simulink model "Resp18e_updatedPulse"  (Simulink 7.3)
settings: Solver=ode23  StartTime=0.0  StopTime=20  FixedStep=0.01  MaxStep=0.05  RelTol=1e-6
values from neighbouring files (symbols this model uses):
  alpha_CO2_brain = 2.9/1e3*760/P_stp/K_stp    (= 0.00097047576489)    [initialize_parameters.m]
  alpha_CO2_fat = 0.9/K_stp/P_stp    (= 0.000396292281489)    [initialize_parameters.m]
  alpha_CO2_heart = 2.4/1e3*760/P_stp/K_stp    (= 0.00080315235715)    [initialize_parameters.m]
  alpha_CO2_lean = 4.2/1e3*760/P_stp/K_stp    (= 0.00140551662501)    [initialize_parameters.m]
  alpha_CO2_lungtiss_fast = alpha_CO2_lungtiss_fast./0.1333    [initialize_parameters.m]
  alpha_CO2_muscle = 4.2/1e3*760/P_stp/K_stp    (= 0.00140551662501)    [initialize_parameters.m]
  alpha_CO2_other = 3.0/1e3*760/P_stp/K_stp    (= 0.00100394044644)    [initialize_parameters.m]
  alpha_O2_fat = 5*0.024/K_stp/P_stp    (= 5.28389708651e-05)    [initialize_parameters.m]
  alpha_O2_tissue = 0.024/K_stp/P_stp    (= 1.0567794173e-05)    [initialize_parameters.m]
  BOHRF0 = O2_SHIFT - T_BLOOD_M_37 * (0.024 + BOHRF * 0.0147) - BOHRF1 * 7.4    (= -3.552)    [initialize_parameters.m]
  BOHRF1 = BOHRF * (1 - T_BLOOD_M_37 * 0.0065)    (= 0.48)    [initialize_parameters.m]
  C_a_CO2_i = 20.8e-3    (= 0.0208)    [initialize_parameters.m]    (also in resp18e_ic_norm.mat = 0.0202734801806)
  C_a_O2_i = 8.95e-3    (= 0.00895)    [initialize_parameters.m]    (also in resp18e_ic_norm.mat = 0.00918087581167)
  CAP_O2 = 0.01 * CAP_O2    (= 0.201)    [initialize_parameters.m]
  Cardiac_duty_cycle = 40    [initialize_parameters.m]
  Co_CO2_brain = 401*K_Co_CO2/1e3/K_stp    (= 0.0107345869894)    [initialize_parameters.m]
  Co_CO2_heart = 487*K_Co_CO2/1e3/K_stp    (= 0.0130367677403)    [initialize_parameters.m]
  Co_CO2_lean = 342*K_Co_CO2/1e3/K_stp    (= 0.00915518391618)    [initialize_parameters.m]
  Co_CO2_muscle = 342*K_Co_CO2/1e3/K_stp    (= 0.00915518391618)    [initialize_parameters.m]
  Co_CO2_other = 355*K_Co_CO2/1e3/K_stp    (= 0.00950318798317)    [initialize_parameters.m]
  DH2ODS = DH2ODS + 0.007 * HB_MEQ * (HB_MEQ - 9) / (13.5 * (13.5 - 9))    (= 0.00498709726946)    [initialize_parameters.m]
  F_insp_alv_alvds = F_v_alv_deadspace / F_insp_hivq    (= 0.00299401197605)    [initialize_parameters.m]
  F_insp_alv_hivq = F_v_alv_hivq      / F_insp_hivq    (= 0.997005988024)    [initialize_parameters.m]
  F_insp_alv_lovq = F_v_alv_lovq      / F_insp_lovq    (= 0.5)    [initialize_parameters.m]
  F_insp_alv_midvq = F_v_alv_midvq     / F_insp_lovq    (= 0.5)    [initialize_parameters.m]
  F_insp_hivq = F_v_alv_deadspace + F_v_alv_hivq    (= 0.334)    [initialize_parameters.m]
  F_insp_lovq = F_v_alv_midvq     + F_v_alv_lovq    (= 0.666)    [initialize_parameters.m]
  Fi_CO2_param_est = 0.01    [initialize_parameters.m]
  Fi_error = 1e-6    (= 1e-06)    [initialize_parameters.m]
  Fi_N2_mean = 1-(Fi_O2_mean + Fi_N2O_mean)    (= 0.65)    [initialize_parameters.m]
  Fi_O2_mean = 0.35    [initialize_parameters.m]
  Fi_O2_param_est = 0.01    [initialize_parameters.m]
  Fq_brain = 0.114    [initialize_parameters.m]
  Fq_error = 1e-8    (= 1e-08)    [initialize_parameters.m]
  Fq_fat = 0.103    [initialize_parameters.m]
  Fq_heart = 0.041    [initialize_parameters.m]
  Fq_hepatic = 0.069    [initialize_parameters.m]
  Fq_kidneys = 0.215    [initialize_parameters.m]
  Fq_lean = 0.090    (= 0.09)    [initialize_parameters.m]
  Fq_lungs_anatomicalshunt = 0.01    [initialize_parameters.m]
  Fq_lungs_hivq = (1-Fq_lungs_pulmshunt-Fq_lungs_anatomicalshunt)    *F_v_alv_hivq/(F_v_alv_hivq+F_v_alv_midvq+F_v_alv_lovq)    (= 0.3)    [initialize_parameters.m]
  Fq_lungs_lovq = (1-Fq_lungs_pulmshunt-Fq_lungs_anatomicalshunt)    *F_v_alv_lovq/(F_v_alv_hivq+F_v_alv_midvq+F_v_alv_lovq)    (= 0.3)    [initialize_parameters.m]
  Fq_lungs_midvq = (1-Fq_lungs_pulmshunt-Fq_lungs_anatomicalshunt)    *F_v_alv_midvq/(F_v_alv_hivq+F_v_alv_midvq+F_v_alv_lovq)    (= 0.3)    [initialize_parameters.m]
  Fq_lungs_pulmshunt = 0.09    [initialize_parameters.m]
  Fq_muscle = 0.096    [initialize_parameters.m]
  Fq_pershunt = 0.101    [initialize_parameters.m]
  Fq_portal = 0.171    [initialize_parameters.m]
  FRC = 2.2    [initialize_parameters.m]
  H2OB = H2OVC + 0.938 * (1 - VC_74)    (= 0.840191964286)    [initialize_parameters.m]
  k_CO2_lungtiss_fast_alvds = k_CO2_lungtiss_fast*F_v_alv_deadspace    (= 3.63090772693e-07)    [initialize_parameters.m]
  k_CO2_lungtiss_fast_hivq = k_CO2_lungtiss_fast*F_v_alv_hivq    (= 0.000120909227307)    [initialize_parameters.m]
  k_CO2_lungtiss_fast_lovq = k_CO2_lungtiss_fast*F_v_alv_lovq    (= 0.000120909227307)    [initialize_parameters.m]
  k_CO2_lungtiss_fast_midvq = k_CO2_lungtiss_fast*F_v_alv_midvq    (= 0.000120909227307)    [initialize_parameters.m]
  k_CO2_lungtiss_slow_alvds = k_CO2_lungtiss_slow*F_v_alv_deadspace    (= 4.95123780945e-09)    [initialize_parameters.m]
  k_CO2_lungtiss_slow_hivq = k_CO2_lungtiss_slow*F_v_alv_hivq    (= 1.64876219055e-06)    [initialize_parameters.m]
  k_CO2_lungtiss_slow_lovq = k_CO2_lungtiss_slow*F_v_alv_lovq    (= 1.64876219055e-06)    [initialize_parameters.m]
  k_CO2_lungtiss_slow_midvq = k_CO2_lungtiss_slow*F_v_alv_midvq    (= 1.64876219055e-06)    [initialize_parameters.m]
  K_diff_CO2_hivq = K_diff_CO2*F_v_alv_hivq    (= 0.0014985)    [initialize_parameters.m]
  K_diff_CO2_lovq = K_diff_CO2*F_v_alv_lovq    (= 0.0014985)    [initialize_parameters.m]
  K_diff_CO2_midvq = K_diff_CO2*F_v_alv_midvq    (= 0.0014985)    [initialize_parameters.m]
  K_diff_O2_hivq = K_diff_O2*F_v_alv_hivq    (= 7.326e-05)    [initialize_parameters.m]
  K_diff_O2_lovq = K_diff_O2*F_v_alv_lovq    (= 7.326e-05)    [initialize_parameters.m]
  K_diff_O2_midvq = K_diff_O2*F_v_alv_midvq    (= 7.326e-05)    [initialize_parameters.m]
  K_exp_alv_alvds = 1/1    (= 1)    [initialize_parameters.m]
  K_exp_alv_hivq = 1/1    (= 1)    [initialize_parameters.m]
  K_press = 760/101.325    (= 7.50061682704)    [initialize_parameters.m]
  K_stp = R*(T_stp+273.15)/(P_stp*1000)    (= 22.4135311621)    [initialize_parameters.m]
  Kg_alv = R*(T_alv+273.15)/(P_baro*1000)    (= 25.3668469802)    [initialize_parameters.m]
  LN10 = 2.30258509299405    (= 2.30258509299)    [initialize_parameters.m]
  m_alv_alvds_i = (FRC-V_deadspace_total)/Kg_alv * F_v_alv_deadspace    [initialize_parameters.m]
  m_alv_hivq_i = (FRC-V_deadspace_total)/Kg_alv * F_v_alv_hivq    [initialize_parameters.m]
  m_alv_lovq_i = (FRC-V_deadspace_total)/Kg_alv * F_v_alv_lovq    [initialize_parameters.m]
  m_alv_midvq_i = (FRC-V_deadspace_total)/Kg_alv * F_v_alv_midvq    [initialize_parameters.m]
  m_CO2_alv_alvds_i = F_CO2_i * m_alv_alvds_i    [initialize_parameters.m]
  m_CO2_alv_hivq_i = F_CO2_i * m_alv_hivq_i    [initialize_parameters.m]
  m_CO2_alv_lovq_i = F_CO2_i * m_alv_lovq_i    [initialize_parameters.m]
  m_CO2_alv_midvq_i = F_CO2_i * m_alv_midvq_i    [initialize_parameters.m]
  m_CO2_brain_b_i = C_a_CO2_i*Vb_brain    (= 0.002184)    [initialize_parameters.m]
  m_CO2_brain_t_i = (Co_CO2_brain  + alpha_CO2_brain *P_v_CO2_i)* Vt_brain    (= 0.0171268217946)    [initialize_parameters.m]
  m_CO2_common_b_i = C_a_CO2_i*Vb_common    (= 0.0170421333333)    [initialize_parameters.m]
  m_CO2_ds0_i = F_CO2_i*m_ds0_i    (= 0.000985538329597)    [initialize_parameters.m]
  m_CO2_ds_large_i = F_CO2_i * m_deadspace_large_1    [initialize_parameters.m]
  m_CO2_ds_med_hivq1_i = F_CO2_i * m_deadspace_med_hivq_1    [initialize_parameters.m]
  m_CO2_ds_med_hivq2_i = F_CO2_i * m_deadspace_med_hivq_2    [initialize_parameters.m]
  m_CO2_ds_med_lovq1_i = F_CO2_i * m_deadspace_med_lovq_1    [initialize_parameters.m]
  m_CO2_ds_med_lovq2_i = F_CO2_i * m_deadspace_med_lovq_2    [initialize_parameters.m]
  m_CO2_ds_small_alvds_i = F_CO2_i * m_deadspace_small_alvdeadspace    [initialize_parameters.m]
  m_CO2_ds_small_hivq_i = F_CO2_i * m_deadspace_small_hivq    [initialize_parameters.m]
  m_CO2_ds_small_lovq_i = F_CO2_i * m_deadspace_small_lovq    [initialize_parameters.m]
  m_CO2_ds_small_midvq_i = F_CO2_i * m_deadspace_small_midvq    [initialize_parameters.m]
  m_CO2_fat_b_i = C_a_CO2_i*Vb_fat    (= 0.0116896)    [initialize_parameters.m]
  m_CO2_fat_t_i = P_a_CO2_i*alpha_CO2_fat*Vt_fat    (= 0.0302752719501)    [initialize_parameters.m]
  m_CO2_heart_b_i = C_a_CO2_i*Vb_heart    (= 0.000832)    [initialize_parameters.m]
  m_CO2_heart_t_i = (Co_CO2_heart  + alpha_CO2_heart *P_v_CO2_i)* Vt_heart    (= 0.00402544335149)    [initialize_parameters.m]
  m_CO2_hepatic_b_i = C_a_CO2_i*Vb_hepatic    (= 0.0019136)    [initialize_parameters.m]
  m_CO2_kidneys_b_i = C_a_CO2_i*Vb_kidneys    (= 0.0012064)    [initialize_parameters.m]
  m_CO2_kidneys_t_i = (Co_CO2_other  + alpha_CO2_other *P_v_CO2_i)* Vt_kidneys    (= 0.0045902552907)    [initialize_parameters.m]
  m_CO2_lean_b_i = C_a_CO2_i*Vb_lean    (= 0.0191984)    [initialize_parameters.m]
  m_CO2_lean_t_i = (Co_CO2_lean   + alpha_CO2_lean  *P_v_CO2_i)* Vt_lean    (= 0.0884995401953)    [initialize_parameters.m]
  m_CO2_liver_t_i = (Co_CO2_other  + alpha_CO2_other *P_v_CO2_i)* Vt_liver    (= 0.0187019339777)    [initialize_parameters.m]
  m_CO2_lungtiss_fast_alvds_i = F_CO2_i*(P_baro-P_A_H2O)*V_lungtiss_alvds *alpha_CO2_lungtiss_fast(2)    [initialize_parameters.m]
  m_CO2_lungtiss_fast_hivq_i = F_CO2_i*(P_baro-P_A_H2O)*V_lungtiss_hivq  *alpha_CO2_lungtiss_fast(2)    [initialize_parameters.m]
  m_CO2_lungtiss_fast_lovq_i = F_CO2_i*(P_baro-P_A_H2O)*V_lungtiss_lovq  *alpha_CO2_lungtiss_fast(2)    [initialize_parameters.m]
  m_CO2_lungtiss_fast_midvq_i = F_CO2_i*(P_baro-P_A_H2O)*V_lungtiss_midvq *alpha_CO2_lungtiss_fast(2)    [initialize_parameters.m]
  m_CO2_lungtiss_slow_alvds_i = F_CO2_i*(P_baro-P_A_H2O)*V_lungtiss_alvds*alpha_CO2_lungtiss_slow    [initialize_parameters.m]
  m_CO2_lungtiss_slow_hivq_i = F_CO2_i*(P_baro-P_A_H2O)*V_lungtiss_hivq *alpha_CO2_lungtiss_slow    [initialize_parameters.m]
  m_CO2_lungtiss_slow_lovq_i = F_CO2_i*(P_baro-P_A_H2O)*V_lungtiss_lovq *alpha_CO2_lungtiss_slow    [initialize_parameters.m]
  m_CO2_lungtiss_slow_midvq_i = F_CO2_i*(P_baro-P_A_H2O)*V_lungtiss_midvq*alpha_CO2_lungtiss_slow    [initialize_parameters.m]
  m_CO2_LV_b_i = C_a_CO2_i*Vb_LV    (= 0.00391733333333)    [initialize_parameters.m]
  m_CO2_muscle_b_i = C_a_CO2_i*Vb_muscle    (= 0.0201344)    [initialize_parameters.m]
  m_CO2_muscle_t_i = (Co_CO2_muscle + alpha_CO2_muscle*P_v_CO2_i)* Vt_muscle    (= 0.363660431061)    [initialize_parameters.m]
  m_CO2_pershunt_b_i = C_a_CO2_i*Vb_pershunt    (= 0.0027248)    [initialize_parameters.m]
  m_CO2_portal_b_i = C_a_CO2_i*Vb_portal    (= 0.0210912)    [initialize_parameters.m]
  m_CO2_portal_t_i = (Co_CO2_other  + alpha_CO2_other *P_v_CO2_i)* Vt_portal    (= 0.0164739329706)    [initialize_parameters.m]
  m_CO2_pulmcap_b_hivq_i = C_a_CO2_i*Vb_pulmcap_hivq    (= 0.000630933333333)    [initialize_parameters.m]
  m_CO2_pulmcap_b_lovq_i = C_a_CO2_i*Vb_pulmcap_lovq    (= 0.000630933333333)    [initialize_parameters.m]
  m_CO2_pulmcap_b_midvq_i = C_a_CO2_i*Vb_pulmcap_midvq    (= 0.000630933333333)    [initialize_parameters.m]
  m_CO2_pulmcap_b_pulmshunt_i = C_a_CO2_i*Vb_pulmcap_pulmshunt    (= 0.0001872)    [initialize_parameters.m]
  m_CO2_RV_b_i = C_v_CO2_i*Vb_RV    (= 0.004181)    [initialize_parameters.m]
  m_N2_alv_alvds_i = Fi_N2_mean * (m_alv_alvds_i - m_CO2_alv_alvds_i)    [initialize_parameters.m]
  ... (+122 more)
undefined symbols (not defined in the file or in its folder): AH2OVC, AHCO3B, DHCO3BDS, litres, mole
libraries: simulink x28
(part 4 of 8)

== system Resp18e_updatedPulse/Patient/Anaesthetic Machine & resp mechanics/Resp PWM ==
  Compare To Constant : simulink/Logic and Bit Operations/Compare To Constant  SystemSampleTime=-1  relop=>=  const=1.0  LogicOutDataTypeMode=boolean  ZeroCross=off
  Compare To Zero : simulink/Logic and Bit Operations/Compare To Zero  SystemSampleTime=-1  relop=<=  LogicOutDataTypeMode=uint8  ZeroCross=off
  Data Type Conversion : DataTypeConversion  OutDataTypeMode=double  OutDataType=fixdt(1, 16)  OutScaling=2^0  OutDataTypeStr=double
  From Workspace : FromWorkspace  VariableName=mod_duty_cycle  SampleTime=0  Interpolate=off  OutputAfterFinalValue=Holding final value
  From Workspace1 : FromWorkspace  VariableName=mod_resp_rate  SampleTime=0  Interpolate=off  OutputAfterFinalValue=Holding final value
  Integrator : Integrator  ExternalReset=rising  UpperSaturationLimit=1  LowerSaturationLimit=0  ZeroCross=off
  Sub : Sum  Inputs=+-  OutDataType=fixdt(1, 16)  OutScaling=2^-10
  Out1 : Outport  OutDataType=fixdt(1, 16)  OutScaling=2^0
  wires:
  From Workspace/1 -> Sub/2
  Integrator/1 -> Compare To Constant/1, Sub/1
  Sub/1 -> Compare To Zero/1
  Compare To Constant/1 -> Integrator/2
  From Workspace1/1 -> Integrator/1
  Data Type Conversion/1 -> Out1/1
  Compare To Zero/1 -> Data Type Conversion/1

== system Resp18e_updatedPulse/Patient/Blood flow distribution control/Pulmonary circulation ==
  Fq_heart : Constant  Value=Fq_lungs_pulmshunt  OutDataType=sfix(16)  OutScaling=2^0
  Fq_heart1 : Constant  Value=Fq_lungs_anatomicalshunt  OutDataType=sfix(16)  OutScaling=2^0
  Fq_heart2 : Constant  Value=Fq_lungs_hivq  OutDataType=sfix(16)  OutScaling=2^0
  Fq_heart3 : Constant  Value=Fq_lungs_lovq  OutDataType=sfix(16)  OutScaling=2^0
  Fq_heart4 : Constant  Value=Fq_lungs_midvq  OutDataType=sfix(16)  OutScaling=2^0
  tag scope: Fq_lungs_anatomicalshunt=global, Fq_lungs_hivq=global, Fq_lungs_lovq=global, Fq_lungs_midvq=global, Fq_lungs_pulmshunt=global
  wires:
  Fq_heart2/1 -> [Fq_lungs_hivq]
  Fq_heart3/1 -> [Fq_lungs_lovq]
  Fq_heart/1 -> [Fq_lungs_pulmshunt]
  Fq_heart1/1 -> [Fq_lungs_anatomicalshunt]
  Fq_heart4/1 -> [Fq_lungs_midvq]

== system Resp18e_updatedPulse/Patient/Blood flow distribution control/Systemic circulation ==
  Fq_heart1 : Constant  Value=Fq_heart  OutDataType=sfix(16)  OutScaling=2^0
  Fq_heart10 : Constant  Value=Fq_fat  OutDataType=sfix(16)  OutScaling=2^0
  Fq_heart2 : Constant  Value=Fq_kidneys  OutDataType=sfix(16)  OutScaling=2^0
  Fq_heart4 : Constant  Value=Fq_hepatic  OutDataType=sfix(16)  OutScaling=2^0
  Fq_heart5 : Constant  Value=Fq_portal  OutDataType=sfix(16)  OutScaling=2^0
  Fq_heart6 : Constant  Value=Fq_brain  OutDataType=sfix(16)  OutScaling=2^0
  Fq_heart7 : Constant  Value=Fq_pershunt  OutDataType=sfix(16)  OutScaling=2^0
  Fq_heart8 : Constant  Value=Fq_muscle  OutDataType=sfix(16)  OutScaling=2^0
  Fq_heart9 : Constant  Value=Fq_lean  OutDataType=sfix(16)  OutScaling=2^0
  tag scope: Fq_brain=global, Fq_fat=global, Fq_heart=global, Fq_hepatic=global, Fq_kidneys=global, Fq_lean=global, Fq_muscle=global, Fq_pershunt=global, Fq_portal=global
  wires:
  Fq_heart2/1 -> [Fq_kidneys]
  Fq_heart4/1 -> [Fq_hepatic]
  Fq_heart5/1 -> [Fq_portal]
  Fq_heart6/1 -> [Fq_brain]
  Fq_heart7/1 -> [Fq_pershunt]
  Fq_heart8/1 -> [Fq_muscle]
  Fq_heart9/1 -> [Fq_lean]
  Fq_heart10/1 -> [Fq_fat]
  Fq_heart1/1 -> [Fq_heart]

== system Resp18e_updatedPulse/Patient/Brain/Brain ==
  note: Note that output vector is C_CO2, C_O2, Fq_heart
  note: NB: Integrators CO2_in and O2_out are purely for mass balance calculations
  note: mole/l
  Ca_gases : Inport  PortDimensions=3  OutDataType=sfix(16)  OutScaling=2^0
  Blood gas curves Olszowka SI Units : Subsystem
  CO2_brain : Integrator  InitialCondition=m_CO2_brain_t_i
  CO2_in : Integrator  InitialConditionSource=external
  C_CO2 body : Gain  Gain=1/Vt_brain  ParameterDataType=sfix(16)  ParameterScaling=2^0  OutDataType=sfix(16)  OutScaling=2^0  SaturateOnIntegerOverflow=on  OutDataTypeStr=Inherit: Same as input  ParamDataTypeStr=Inherit: Same as input
  C_CO2 body1 : Gain  Gain=1/Vt_brain  ParameterDataType=sfix(16)  ParameterScaling=2^0  OutDataType=sfix(16)  OutScaling=2^0  SaturateOnIntegerOverflow=on  OutDataTypeStr=Inherit: Same as input  ParamDataTypeStr=Inherit: Same as input
  C_CO2 body2 : Gain  Gain=-1  ParameterDataType=sfix(16)  ParameterScaling=2^0  OutDataType=sfix(16)  OutScaling=2^0  SaturateOnIntegerOverflow=on  OutDataTypeStr=Inherit: Same as input  ParamDataTypeStr=Inherit: Same as input
  Constant : Constant  Value=0  OutDataType=sfix(16)  OutScaling=2^0
  Constant1 : Constant  Value=0  OutDataType=sfix(16)  OutScaling=2^0
  Demux : Demux  Outputs=3
  InvTissue diss curves : Subsystem
  Mux : Mux  Inputs=3
  O2_brain : Integrator  InitialCondition=m_O2_brain_t_i
  O2_out : Integrator  InitialConditionSource=external
  P4 : Product  Inputs=**  OutDataType=sfix(16)  OutScaling=2^0  SaturateOnIntegerOverflow=on  RndMeth=Zero  InputSameDT=on  OutDataTypeStr=Inherit: Same as first input
  P5 : Product  Inputs=**  OutDataType=sfix(16)  OutScaling=2^0  SaturateOnIntegerOverflow=on  RndMeth=Zero  InputSameDT=on  OutDataTypeStr=Inherit: Same as first input
  P6 : Product  Inputs=**  OutDataType=sfix(16)  OutScaling=2^0  SaturateOnIntegerOverflow=on  RndMeth=Zero  InputSameDT=on  OutDataTypeStr=Inherit: Same as first input
  P_baro1 : Constant  Value=mdot_CO2_brain  OutDataType=sfix(16)  OutScaling=2^0
  P_baro2 : Constant  Value=mdot_O2_brain  OutDataType=sfix(16)  OutScaling=2^0
  Terminator : Terminator
  Terminator1 : Terminator
  Tidal vol2 : Sum  Inputs=-+  OutDataType=sfix(16)  OutScaling=2^0  SaturateOnIntegerOverflow=on  InputSameDT=on  OutDataTypeStr=Inherit: Same as first input
  Tidal vol3 : Sum  Inputs=+-  OutDataType=sfix(16)  OutScaling=2^0  SaturateOnIntegerOverflow=on  InputSameDT=on  OutDataTypeStr=Inherit: Same as first input
  Tidal vol4 : Sum  OutDataType=sfix(16)  OutScaling=2^0  SaturateOnIntegerOverflow=on  InputSameDT=on  OutDataTypeStr=Inherit: Same as first input
  Tidal vol5 : Sum  Inputs=+-  OutDataType=sfix(16)  OutScaling=2^0  SaturateOnIntegerOverflow=on  InputSameDT=on  OutDataTypeStr=Inherit: Same as first input
  To Workspace1 : ToWorkspace  VariableName=C_v_O2_brain  SampleTime=t_sample  SaveFormat=Array
  To Workspace2 : ToWorkspace  VariableName=C_v_CO2_brain  SampleTime=t_sample  SaveFormat=Array
  Cv_gases : Outport  OutDataType=sfix(16)  OutScaling=2^0
  wires:
  Demux/3 -> Mux/3, P6/2
  InvTissue diss curves/2(PT_O2) -> Blood gas curves Olszowka SI Units/2(P_O2)
  InvTissue diss curves/1(PT_CO2) -> Blood gas curves Olszowka SI Units/1(P_CO2)
  CO2_brain/1 -> C_CO2 body/1
  O2_brain/1 -> C_CO2 body1/1
  [Qpdot] -> P6/1
  P6/1 -> P4/1, P5/1
  Tidal vol5/1 -> O2_brain/1
  P5/1 -> Tidal vol5/1
  P4/1 -> Tidal vol4/2
  Tidal vol4/1 -> CO2_brain/1
  Tidal vol3/1 -> P5/2
  Tidal vol2/1 -> P4/2
  C_CO2 body1/1 -> InvTissue diss curves/2(C_O2)
  C_CO2 body/1 -> InvTissue diss curves/1(C_CO2)
  P_baro1/1 -> Tidal vol4/1, C_CO2 body2/1
  C_CO2 body2/1 -> CO2_in/1
  CO2_in/1 -> Terminator/1
  P_baro2/1 -> Tidal vol5/2, O2_out/1
  O2_out/1 -> Terminator1/1
  Ca_gases/1 -> Demux/1
  Demux/1 -> Tidal vol2/2
  Demux/2 -> Tidal vol3/1
  Mux/1 -> Cv_gases/1
  Blood gas curves Olszowka SI Units/2(C_O2) -> Mux/2, Tidal vol3/2, To Workspace1/1
  Blood gas curves Olszowka SI Units/1(C_CO2) -> Mux/1, Tidal vol2/1, To Workspace2/1
  Constant1/1 -> CO2_in/2
  Constant/1 -> O2_out/2

== system Resp18e_updatedPulse/Patient/Brain/Delay_brain ==
  note: This block performs the following functions:
      | 1. Keeps a record of the quantity of CO2 in aorta
      | 2.  Keeps a record of the quantity of O2 in aorta
      | 3. Delays C_CO2 and C_O2 signals by a time
      | proportional to the aortic volume and inversely
      | proportional to Qpdot.
      | 4. Outputs are delayed C_CO2 and C_O2 signals (moles/l)
      | NB: This subsystem cannot handle varying Qpdot
  note: Constant Qpdot only
  C_gases : Inport  PortDimensions=2  OutDataType=sfix(16)  OutScaling=2^0
  CO2 O2 : Demux  Outputs=2
  CO2 xport delay : VariableTransportDelay  MaximumDelay=20  InitialOutput=C_a_CO2_i  MaximumPoints=n_delay_buffer
  CO2_d : Integrator  InitialCondition=m_CO2_brain_b_i
  Fixed delay : Fcn  Expr=Vb_brain/u(1)
  Mux : Mux  Inputs=3
  O2 delay : VariableTransportDelay  MaximumDelay=20  InitialOutput=C_a_O2_i  MaximumPoints=n_delay_buffer
  O2_d : Integrator  InitialCondition=m_O2_brain_b_i
  Product{1..5} (5 alike) : Product  OutDataType=sfix(16)  OutScaling=2^0  SaturateOnIntegerOverflow=on  RndMeth=Zero  InputSameDT=on  OutDataTypeStr=Inherit: Same as first input
  Terminator : Terminator
  Terminator1 : Terminator
  Tidal vol2 : Sum  Inputs=+-  OutDataType=sfix(16)  OutScaling=2^0  SaturateOnIntegerOverflow=on  InputSameDT=on  OutDataTypeStr=Inherit: Same as first input
  Tidal vol3 : Sum  Inputs=+-  OutDataType=sfix(16)  OutScaling=2^0  SaturateOnIntegerOverflow=on  InputSameDT=on  OutDataTypeStr=Inherit: Same as first input
  Ca_gases_d : Outport  OutDataType=sfix(16)  OutScaling=2^0
  wires:
  [Fq_brain] -> Mux/3, Product5/2
  CO2_d/1 -> Terminator1/1
  Fixed delay/1 -> CO2 xport delay/2, O2 delay/2
  Tidal vol2/1 -> CO2_d/1
  Product1/1 -> Tidal vol2/1
  Tidal vol3/1 -> O2_d/1
  Product4/1 -> Tidal vol3/1
  O2_d/1 -> Terminator/1
  CO2 xport delay/1 -> Mux/1, Product2/1
  O2 delay/1 -> Mux/2, Product3/2
  Product3/1 -> Tidal vol3/2
  Product2/1 -> Tidal vol2/2
  CO2 O2/1 -> Product1/1, CO2 xport delay/1
  C_gases/1 -> CO2 O2/1
  CO2 O2/2 -> O2 delay/1, Product4/2
  Mux/1 -> Ca_gases_d/1
  [Qpdot] -> Product5/1
  Product5/1 -> Fixed delay/1, Product1/2, Product3/1, Product4/1, Product2/2

== system Resp18e_updatedPulse/Patient/Fat/Delay_fat ==
  note: Constant Qpdot only
  note: This block performs the following functions:
      | 1. Keeps a record of the quantity of CO2 in aorta
      | 2.  Keeps a record of the quantity of O2 in aorta
      | 3. Delays C_CO2 and C_O2 signals by a time
      | proportional to the aortic volume and inversely
      | proportional to Qpdot.
      | 4. Outputs are delayed C_CO2 and C_O2 signals (moles/l)
      | NB: This subsystem cannot handle varying Qpdot
  C_gases : Inport  PortDimensions=2  OutDataType=sfix(16)  OutScaling=2^0
  CO2 O2 : Demux  Outputs=2
  CO2 delay : VariableTransportDelay  MaximumDelay=200  InitialOutput=C_a_CO2_i  MaximumPoints=n_delay_buffer
  CO2_d : Integrator  InitialCondition=m_CO2_fat_b_i
  Fixed delay : Fcn  Expr=Vb_fat/u(1)
  Mux : Mux  Inputs=3
  O2 delay : VariableTransportDelay  MaximumDelay=200  InitialOutput=C_a_O2_i  MaximumPoints=n_delay_buffer
  O2_d : Integrator  InitialCondition=m_O2_fat_b_i
  Product{1..5} (5 alike) : Product  OutDataType=sfix(16)  OutScaling=2^0  SaturateOnIntegerOverflow=on  RndMeth=Zero  InputSameDT=on  OutDataTypeStr=Inherit: Same as first input
  Terminator : Terminator
  Terminator1 : Terminator
  Tidal vol2 : Sum  Inputs=+-  OutDataType=sfix(16)  OutScaling=2^0  SaturateOnIntegerOverflow=on  InputSameDT=on  OutDataTypeStr=Inherit: Same as first input
  Tidal vol3 : Sum  Inputs=+-  OutDataType=sfix(16)  OutScaling=2^0  SaturateOnIntegerOverflow=on  InputSameDT=on  OutDataTypeStr=Inherit: Same as first input
  Ca_gases_d : Outport  OutDataType=sfix(16)  OutScaling=2^0
  wires:
  Product5/1 -> Product2/2, Product4/1, Product3/1, Product1/2, Fixed delay/1
  [Qpdot] -> Product5/1
  Mux/1 -> Ca_gases_d/1
  CO2 O2/2 -> Product4/2, O2 delay/1
  C_gases/1 -> CO2 O2/1
  CO2 O2/1 -> CO2 delay/1, Product1/1
  Product2/1 -> Tidal vol2/2
  Product3/1 -> Tidal vol3/2
  O2 delay/1 -> Product3/2, Mux/2
  CO2 delay/1 -> Product2/1, Mux/1
  O2_d/1 -> Terminator/1
  Product4/1 -> Tidal vol3/1
  Tidal vol3/1 -> O2_d/1
  Product1/1 -> Tidal vol2/1
  Tidal vol2/1 -> CO2_d/1
  Fixed delay/1 -> O2 delay/2, CO2 delay/2
  CO2_d/1 -> Terminator1/1
  [Fq_fat] -> Product5/2, Mux/3

== system Resp18e_updatedPulse/Patient/Fat/fat ==
  note: mole/l
  note: NB: Integrators CO2_in and O2_out are purely for mass balance calculations
  note: Note that output vector is C_CO2, C_O2, Fq_heart
  Ca_gases : Inport  PortDimensions=3  OutDataType=sfix(16)  OutScaling=2^0
  Blood gas curves Olszowka SI Units : Subsystem
  CO2_fat : Integrator  InitialCondition=m_CO2_fat_t_i
  CO2_in : Integrator  InitialConditionSource=external
  C_CO2 body : Gain  Gain=1/Vt_fat  ParameterDataType=sfix(16)  ParameterScaling=2^0  OutDataType=sfix(16)  OutScaling=2^0  SaturateOnIntegerOverflow=on  OutDataTypeStr=Inherit: Same as input  ParamDataTypeStr=Inherit: Same as input
  C_CO2 body1 : Gain  Gain=1/Vt_fat  ParameterDataType=sfix(16)  ParameterScaling=2^0  OutDataType=sfix(16)  OutScaling=2^0  SaturateOnIntegerOverflow=on  OutDataTypeStr=Inherit: Same as input  ParamDataTypeStr=Inherit: Same as input
  C_CO2 body2 : Gain  Gain=-1  ParameterDataType=sfix(16)  ParameterScaling=2^0  OutDataType=sfix(16)  OutScaling=2^0  SaturateOnIntegerOverflow=on  OutDataTypeStr=Inherit: Same as input  ParamDataTypeStr=Inherit: Same as input
  Constant : Constant  Value=0  OutDataType=sfix(16)  OutScaling=2^0
  Constant1 : Constant  Value=0  OutDataType=sfix(16)  OutScaling=2^0
  Demux : Demux  Outputs=3
  Inv fat diss curves : Subsystem
  Mux : Mux  Inputs=3
  O2_fat : Integrator  InitialCondition=m_O2_fat_t_i
  O2_out : Integrator  InitialConditionSource=external
  P4 : Product  Inputs=**  OutDataType=sfix(16)  OutScaling=2^0  SaturateOnIntegerOverflow=on  RndMeth=Zero  InputSameDT=on  OutDataTypeStr=Inherit: Same as first input
  P5 : Product  Inputs=**  OutDataType=sfix(16)  OutScaling=2^0  SaturateOnIntegerOverflow=on  RndMeth=Zero  InputSameDT=on  OutDataTypeStr=Inherit: Same as first input
  P6 : Product  Inputs=**  OutDataType=sfix(16)  OutScaling=2^0  SaturateOnIntegerOverflow=on  RndMeth=Zero  InputSameDT=on  OutDataTypeStr=Inherit: Same as first input
  P_baro1 : Constant  Value=mdot_CO2_fat  OutDataType=sfix(16)  OutScaling=2^0
  P_baro2 : Constant  Value=mdot_O2_fat  OutDataType=sfix(16)  OutScaling=2^0
  Terminator : Terminator
  Terminator1 : Terminator
  Tidal vol2 : Sum  Inputs=-+  OutDataType=sfix(16)  OutScaling=2^0  SaturateOnIntegerOverflow=on  InputSameDT=on  OutDataTypeStr=Inherit: Same as first input
  Tidal vol3 : Sum  Inputs=+-  OutDataType=sfix(16)  OutScaling=2^0  SaturateOnIntegerOverflow=on  InputSameDT=on  OutDataTypeStr=Inherit: Same as first input
  Tidal vol4 : Sum  OutDataType=sfix(16)  OutScaling=2^0  SaturateOnIntegerOverflow=on  InputSameDT=on  OutDataTypeStr=Inherit: Same as first input
  Tidal vol5 : Sum  Inputs=+-  OutDataType=sfix(16)  OutScaling=2^0  SaturateOnIntegerOverflow=on  InputSameDT=on  OutDataTypeStr=Inherit: Same as first input
  To Workspace2 : ToWorkspace  VariableName=C_v_CO2_fat  SampleTime=t_sample  SaveFormat=Array
  To Workspace3 : ToWorkspace  VariableName=C_v_O2_fat  SampleTime=t_sample  SaveFormat=Array
  Cv_gases : Outport  OutDataType=sfix(16)  OutScaling=2^0
  wires:
  Blood gas curves Olszowka SI Units/1(C_CO2) -> Mux/1, Tidal vol2/1, To Workspace2/1
  Blood gas curves Olszowka SI Units/2(C_O2) -> Mux/2, Tidal vol3/2, To Workspace3/1
  Mux/1 -> Cv_gases/1
  Demux/2 -> Tidal vol3/1
  Demux/1 -> Tidal vol2/2
  Ca_gases/1 -> Demux/1
  O2_out/1 -> Terminator1/1
  P_baro2/1 -> O2_out/1, Tidal vol5/2
  CO2_in/1 -> Terminator/1
  C_CO2 body2/1 -> CO2_in/1
  P_baro1/1 -> C_CO2 body2/1, Tidal vol4/1
  C_CO2 body/1 -> Inv fat diss curves/1(C_CO2)
  C_CO2 body1/1 -> Inv fat diss curves/2(C_O2)
  Tidal vol2/1 -> P4/2
  Tidal vol3/1 -> P5/2
  Tidal vol4/1 -> CO2_fat/1
  P4/1 -> Tidal vol4/2
  P5/1 -> Tidal vol5/1
  Tidal vol5/1 -> O2_fat/1
  P6/1 -> P5/1, P4/1
  [Qpdot] -> P6/1
  O2_fat/1 -> C_CO2 body1/1
  CO2_fat/1 -> C_CO2 body/1
  Inv fat diss curves/1(P_CO2) -> Blood gas curves Olszowka SI Units/1(P_CO2)
  Inv fat diss curves/2(P_O2) -> Blood gas curves Olszowka SI Units/2(P_O2)
  Demux/3 -> P6/2, Mux/3
  Constant/1 -> CO2_in/2
  Constant1/1 -> O2_out/2

== system Resp18e_updatedPulse/Patient/Heart/Delay_heart ==
  note: Constant Qpdot only
  note: This block performs the following functions:
      | 1. Keeps a record of the quantity of CO2 in aorta
      | 2.  Keeps a record of the quantity of O2 in aorta
      | 3. Delays C_CO2 and C_O2 signals by a time
      | proportional to the aortic volume and inversely
      | proportional to Qpdot.
      | 4. Outputs are delayed C_CO2 and C_O2 signals (moles/l)
      | NB: This subsystem cannot handle varying Qpdot
  C_gases : Inport  PortDimensions=2  OutDataType=sfix(16)  OutScaling=2^0
  CO2 O2 : Demux  Outputs=2
  CO2 xport delay : VariableTransportDelay  MaximumDelay=20  InitialOutput=C_a_CO2_i  MaximumPoints=n_delay_buffer
  CO2_d : Integrator  InitialCondition=m_CO2_heart_b_i
  Fixed delay : Fcn  Expr=Vb_heart/u(1)
  Mux : Mux  Inputs=3
  O2 delay : VariableTransportDelay  MaximumDelay=20  InitialOutput=C_a_O2_i  MaximumPoints=n_delay_buffer
  O2_d : Integrator  InitialCondition=m_O2_heart_b_i
  Product{1..5} (5 alike) : Product  OutDataType=sfix(16)  OutScaling=2^0  SaturateOnIntegerOverflow=on  RndMeth=Zero  InputSameDT=on  OutDataTypeStr=Inherit: Same as first input
  Terminator : Terminator
  Terminator1 : Terminator
  Tidal vol2 : Sum  Inputs=+-  OutDataType=sfix(16)  OutScaling=2^0  SaturateOnIntegerOverflow=on  InputSameDT=on  OutDataTypeStr=Inherit: Same as first input
  Tidal vol3 : Sum  Inputs=+-  OutDataType=sfix(16)  OutScaling=2^0  SaturateOnIntegerOverflow=on  InputSameDT=on  OutDataTypeStr=Inherit: Same as first input
  Ca_gases_d : Outport  OutDataType=sfix(16)  OutScaling=2^0
  wires:
  Product5/1 -> Product2/2, Product4/1, Product3/1, Product1/2, Fixed delay/1
  [Qpdot] -> Product5/1
  Mux/1 -> Ca_gases_d/1
  CO2 O2/2 -> Product4/2, O2 delay/1
  C_gases/1 -> CO2 O2/1
  CO2 O2/1 -> CO2 xport delay/1, Product1/1
  Product2/1 -> Tidal vol2/2
  Product3/1 -> Tidal vol3/2
  O2 delay/1 -> Product3/2, Mux/2
  CO2 xport delay/1 -> Product2/1, Mux/1
  O2_d/1 -> Terminator/1
  Product4/1 -> Tidal vol3/1
  Tidal vol3/1 -> O2_d/1
  Product1/1 -> Tidal vol2/1
  Tidal vol2/1 -> CO2_d/1
  Fixed delay/1 -> O2 delay/2, CO2 xport delay/2
  CO2_d/1 -> Terminator1/1
  [Fq_heart] -> Product5/2, Mux/3

== system Resp18e_updatedPulse/Patient/Heart/Heart ==
  note: mole/l
  note: NB: Integrators CO2_in and O2_out are purely for mass balance calculations
  note: Note that output vector is C_CO2, C_O2, Fq_heart
  Ca_gases : Inport  PortDimensions=3  OutDataType=sfix(16)  OutScaling=2^0
  Blood gas curves Olszowka SI Units : Subsystem
  CO2_heart : Integrator  InitialCondition=m_CO2_heart_t_i
  CO2_in : Integrator  InitialConditionSource=external
  C_CO2 body : Gain  Gain=1/Vt_heart  ParameterDataType=sfix(16)  ParameterScaling=2^0  OutDataType=sfix(16)  OutScaling=2^0  SaturateOnIntegerOverflow=on  OutDataTypeStr=Inherit: Same as input  ParamDataTypeStr=Inherit: Same as input
  C_CO2 body1 : Gain  Gain=1/Vt_heart  ParameterDataType=sfix(16)  ParameterScaling=2^0  OutDataType=sfix(16)  OutScaling=2^0  SaturateOnIntegerOverflow=on  OutDataTypeStr=Inherit: Same as input  ParamDataTypeStr=Inherit: Same as input
  C_CO2 body2 : Gain  Gain=-1  ParameterDataType=sfix(16)  ParameterScaling=2^0  OutDataType=sfix(16)  OutScaling=2^0  SaturateOnIntegerOverflow=on  OutDataTypeStr=Inherit: Same as input  ParamDataTypeStr=Inherit: Same as input
  Constant : Constant  Value=0  OutDataType=sfix(16)  OutScaling=2^0
  Constant1 : Constant  Value=0  OutDataType=sfix(16)  OutScaling=2^0
  Demux : Demux  Outputs=3
  InvTissue diss curves : Subsystem
  Mux : Mux  Inputs=3
  O2_heart : Integrator  InitialCondition=m_O2_heart_t_i
  O2_out : Integrator  InitialConditionSource=external
  P4 : Product  Inputs=**  OutDataType=sfix(16)  OutScaling=2^0  SaturateOnIntegerOverflow=on  RndMeth=Zero  InputSameDT=on  OutDataTypeStr=Inherit: Same as first input
  P5 : Product  Inputs=**  OutDataType=sfix(16)  OutScaling=2^0  SaturateOnIntegerOverflow=on  RndMeth=Zero  InputSameDT=on  OutDataTypeStr=Inherit: Same as first input
  P6 : Product  Inputs=**  OutDataType=sfix(16)  OutScaling=2^0  SaturateOnIntegerOverflow=on  RndMeth=Zero  InputSameDT=on  OutDataTypeStr=Inherit: Same as first input
  P_baro1 : Constant  Value=mdot_CO2_heart  OutDataType=sfix(16)  OutScaling=2^0
  P_baro2 : Constant  Value=mdot_O2_heart  OutDataType=sfix(16)  OutScaling=2^0
  Terminator : Terminator
  Terminator1 : Terminator
  Tidal vol2 : Sum  Inputs=-+  OutDataType=sfix(16)  OutScaling=2^0  SaturateOnIntegerOverflow=on  InputSameDT=on  OutDataTypeStr=Inherit: Same as first input
  Tidal vol3 : Sum  Inputs=+-  OutDataType=sfix(16)  OutScaling=2^0  SaturateOnIntegerOverflow=on  InputSameDT=on  OutDataTypeStr=Inherit: Same as first input
  Tidal vol4 : Sum  OutDataType=sfix(16)  OutScaling=2^0  SaturateOnIntegerOverflow=on  InputSameDT=on  OutDataTypeStr=Inherit: Same as first input
  Tidal vol5 : Sum  Inputs=+-  OutDataType=sfix(16)  OutScaling=2^0  SaturateOnIntegerOverflow=on  InputSameDT=on  OutDataTypeStr=Inherit: Same as first input
  To Workspace1 : ToWorkspace  VariableName=C_v_CO2_heart  SampleTime=t_sample  SaveFormat=Array
  To Workspace2 : ToWorkspace  VariableName=C_v_O2_heart  SampleTime=t_sample  SaveFormat=Array
  Cv_gases : Outport  OutDataType=sfix(16)  OutScaling=2^0
  wires:
  Blood gas curves Olszowka SI Units/1(C_CO2) -> Mux/1, Tidal vol2/1, To Workspace1/1
  Blood gas curves Olszowka SI Units/2(C_O2) -> Mux/2, Tidal vol3/2, To Workspace2/1
  Mux/1 -> Cv_gases/1
  Demux/2 -> Tidal vol3/1
  Demux/1 -> Tidal vol2/2
  Ca_gases/1 -> Demux/1
  O2_out/1 -> Terminator1/1
  P_baro2/1 -> O2_out/1, Tidal vol5/2
  CO2_in/1 -> Terminator/1
  C_CO2 body2/1 -> CO2_in/1
  P_baro1/1 -> C_CO2 body2/1, Tidal vol4/1
  C_CO2 body/1 -> InvTissue diss curves/1(C_CO2)
  C_CO2 body1/1 -> InvTissue diss curves/2(C_O2)
  Tidal vol2/1 -> P4/2
  Tidal vol3/1 -> P5/2
  Tidal vol4/1 -> CO2_heart/1
  P4/1 -> Tidal vol4/2
  P5/1 -> Tidal vol5/1
  Tidal vol5/1 -> O2_heart/1
  P6/1 -> P5/1, P4/1
  [Qpdot] -> P6/1
  O2_heart/1 -> C_CO2 body1/1
  CO2_heart/1 -> C_CO2 body/1
  InvTissue diss curves/1(PT_CO2) -> Blood gas curves Olszowka SI Units/1(P_CO2)
  InvTissue diss curves/2(PT_O2) -> Blood gas curves Olszowka SI Units/2(P_O2)
  Demux/3 -> P6/2, Mux/3
  Constant/1 -> O2_out/2
  Constant1/1 -> CO2_in/2

== system Resp18e_updatedPulse/Patient/Kidneys/Delay_kidneys ==
  note: This block performs the following functions:
      | 1. Keeps a record of the quantity of CO2 in aorta
      | 2.  Keeps a record of the quantity of O2 in aorta
      | 3. Delays C_CO2 and C_O2 signals by a time
      | proportional to the aortic volume and inversely
      | proportional to Qpdot.
      | 4. Outputs are delayed C_CO2 and C_O2 signals (moles/l)
      | NB: This subsystem cannot handle varying Qpdot
  note: Constant Qpdot only
  C_gases : Inport  PortDimensions=2  OutDataType=sfix(16)  OutScaling=2^0
  CO2 O2 : Demux  Outputs=2
  CO2 delay : VariableTransportDelay  MaximumDelay=20  InitialOutput=C_a_CO2_i  MaximumPoints=n_delay_buffer
  CO2_d : Integrator  InitialCondition=m_CO2_kidneys_b_i
  Fixed delay : Fcn  Expr=Vb_kidneys/u(1)
  Mux : Mux  Inputs=3
  O2 delay : VariableTransportDelay  MaximumDelay=20  InitialOutput=C_a_O2_i  MaximumPoints=n_delay_buffer
  O2_d : Integrator  InitialCondition=m_O2_kidneys_b_i
  Product{1..5} (5 alike) : Product  OutDataType=sfix(16)  OutScaling=2^0  SaturateOnIntegerOverflow=on  RndMeth=Zero  InputSameDT=on  OutDataTypeStr=Inherit: Same as first input
  Terminator : Terminator
  Terminator1 : Terminator
  Tidal vol2 : Sum  Inputs=+-  OutDataType=sfix(16)  OutScaling=2^0  SaturateOnIntegerOverflow=on  InputSameDT=on  OutDataTypeStr=Inherit: Same as first input
  Tidal vol3 : Sum  Inputs=+-  OutDataType=sfix(16)  OutScaling=2^0  SaturateOnIntegerOverflow=on  InputSameDT=on  OutDataTypeStr=Inherit: Same as first input
  Ca_gases_d : Outport  OutDataType=sfix(16)  OutScaling=2^0
  wires:
  [Fq_kidneys] -> Mux/3, Product5/2
  CO2_d/1 -> Terminator1/1
  Fixed delay/1 -> CO2 delay/2, O2 delay/2
  Tidal vol2/1 -> CO2_d/1
  Product1/1 -> Tidal vol2/1
  Tidal vol3/1 -> O2_d/1
  Product4/1 -> Tidal vol3/1
  O2_d/1 -> Terminator/1
  CO2 delay/1 -> Mux/1, Product2/1
  O2 delay/1 -> Mux/2, Product3/2
  Product3/1 -> Tidal vol3/2
  Product2/1 -> Tidal vol2/2
  CO2 O2/1 -> Product1/1, CO2 delay/1
  C_gases/1 -> CO2 O2/1
  CO2 O2/2 -> O2 delay/1, Product4/2
  Mux/1 -> Ca_gases_d/1
  [Qpdot] -> Product5/1
  Product5/1 -> Fixed delay/1, Product1/2, Product3/1, Product4/1, Product2/2

== system Resp18e_updatedPulse/Patient/Kidneys/Kidneys ==
  note: Note that output vector is C_CO2, C_O2, Fq_heart
  note: NB: Integrators CO2_in and O2_out are purely for mass balance calculations
  note: mole/l
  Ca_gases : Inport  PortDimensions=3  OutDataType=sfix(16)  OutScaling=2^0
  Blood gas curves Olszowka SI Units : Subsystem
  CO2_in : Integrator  InitialConditionSource=external
  CO2_kidneys : Integrator  InitialCondition=m_CO2_kidneys_t_i
  C_CO2 body : Gain  Gain=1/Vt_kidneys  ParameterDataType=sfix(16)  ParameterScaling=2^0  OutDataType=sfix(16)  OutScaling=2^0  SaturateOnIntegerOverflow=on  OutDataTypeStr=Inherit: Same as input  ParamDataTypeStr=Inherit: Same as input
  C_CO2 body1 : Gain  Gain=1/Vt_kidneys  ParameterDataType=sfix(16)  ParameterScaling=2^0  OutDataType=sfix(16)  OutScaling=2^0  SaturateOnIntegerOverflow=on  OutDataTypeStr=Inherit: Same as input  ParamDataTypeStr=Inherit: Same as input
  C_CO2 body2 : Gain  Gain=-1  ParameterDataType=sfix(16)  ParameterScaling=2^0  OutDataType=sfix(16)  OutScaling=2^0  SaturateOnIntegerOverflow=on  OutDataTypeStr=Inherit: Same as input  ParamDataTypeStr=Inherit: Same as input
  Constant : Constant  Value=0  OutDataType=sfix(16)  OutScaling=2^0
  Constant1 : Constant  Value=0  OutDataType=sfix(16)  OutScaling=2^0
  Demux : Demux  Outputs=3
  InvTissue diss curves : Subsystem
  Mux : Mux  Inputs=3
  O2_kidneys : Integrator  InitialCondition=m_O2_kidneys_t_i
  O2_out : Integrator  InitialConditionSource=external
  P4 : Product  Inputs=**  OutDataType=sfix(16)  OutScaling=2^0  SaturateOnIntegerOverflow=on  RndMeth=Zero  InputSameDT=on  OutDataTypeStr=Inherit: Same as first input
  P5 : Product  Inputs=**  OutDataType=sfix(16)  OutScaling=2^0  SaturateOnIntegerOverflow=on  RndMeth=Zero  InputSameDT=on  OutDataTypeStr=Inherit: Same as first input
  P6 : Product  Inputs=**  OutDataType=sfix(16)  OutScaling=2^0  SaturateOnIntegerOverflow=on  RndMeth=Zero  InputSameDT=on  OutDataTypeStr=Inherit: Same as first input
  P_baro1 : Constant  Value=mdot_CO2_kidneys  OutDataType=sfix(16)  OutScaling=2^0
  P_baro2 : Constant  Value=mdot_O2_kidneys  OutDataType=sfix(16)  OutScaling=2^0
  Terminator : Terminator
  Terminator1 : Terminator
  Tidal vol2 : Sum  Inputs=-+  OutDataType=sfix(16)  OutScaling=2^0  SaturateOnIntegerOverflow=on  InputSameDT=on  OutDataTypeStr=Inherit: Same as first input
  Tidal vol3 : Sum  Inputs=+-  OutDataType=sfix(16)  OutScaling=2^0  SaturateOnIntegerOverflow=on  InputSameDT=on  OutDataTypeStr=Inherit: Same as first input
  Tidal vol4 : Sum  OutDataType=sfix(16)  OutScaling=2^0  SaturateOnIntegerOverflow=on  InputSameDT=on  OutDataTypeStr=Inherit: Same as first input
  Tidal vol5 : Sum  Inputs=+-  OutDataType=sfix(16)  OutScaling=2^0  SaturateOnIntegerOverflow=on  InputSameDT=on  OutDataTypeStr=Inherit: Same as first input
  To Workspace2 : ToWorkspace  VariableName=C_v_CO2_kidneys  SampleTime=t_sample  SaveFormat=Array
  To Workspace3 : ToWorkspace  VariableName=C_v_O2_kidneys  SampleTime=t_sample  SaveFormat=Array
  Cv_gases : Outport  OutDataType=sfix(16)  OutScaling=2^0
  wires:
  Demux/3 -> Mux/3, P6/2
  InvTissue diss curves/2(P_O2) -> Blood gas curves Olszowka SI Units/2(P_O2)
  InvTissue diss curves/1(P_CO2) -> Blood gas curves Olszowka SI Units/1(P_CO2)
  CO2_kidneys/1 -> C_CO2 body/1
  O2_kidneys/1 -> C_CO2 body1/1
  [Qpdot] -> P6/1
  P6/1 -> P4/1, P5/1
  Tidal vol5/1 -> O2_kidneys/1
  P5/1 -> Tidal vol5/1
  P4/1 -> Tidal vol4/2
  Tidal vol4/1 -> CO2_kidneys/1
  Tidal vol3/1 -> P5/2
  Tidal vol2/1 -> P4/2
  C_CO2 body1/1 -> InvTissue diss curves/2(C_O2)
  C_CO2 body/1 -> InvTissue diss curves/1(C_CO2)
  P_baro1/1 -> Tidal vol4/1, C_CO2 body2/1
  C_CO2 body2/1 -> CO2_in/1
  CO2_in/1 -> Terminator/1
  P_baro2/1 -> Tidal vol5/2, O2_out/1
  O2_out/1 -> Terminator1/1
  Ca_gases/1 -> Demux/1
  Demux/1 -> Tidal vol2/2
  Demux/2 -> Tidal vol3/1
  Mux/1 -> Cv_gases/1
  Blood gas curves Olszowka SI Units/2(C_O2) -> Mux/2, Tidal vol3/2, To Workspace3/1
  Blood gas curves Olszowka SI Units/1(C_CO2) -> Mux/1, Tidal vol2/1, To Workspace2/1
  Constant/1 -> CO2_in/2
  Constant1/1 -> O2_out/2

== system Resp18e_updatedPulse/Patient/LV + Aorta/Arterial blood gas measurements ==
  note: Arterial blood gase measurements
  C_a_gases : Inport  OutDataType=sfix(16)  OutScaling=2^0
  Demux1 : Demux  Outputs=2
  Olszowka SI units : Subsystem
  To Workspace11 : ToWorkspace  VariableName=pH_a  SampleTime=t_sample  SaveFormat=Array
  To Workspace12 : ToWorkspace  VariableName=P_a_O2  SampleTime=t_sample  SaveFormat=Array
  To Workspace13 : ToWorkspace  VariableName=P_a_CO2  SampleTime=t_sample  SaveFormat=Array
  To Workspace14 : ToWorkspace  VariableName=C_a_CO2  SampleTime=t_sample  SaveFormat=Array
  To Workspace15 : ToWorkspace  VariableName=C_a_O2  SampleTime=t_sample  SaveFormat=Array
  To Workspace16 : ToWorkspace  VariableName=Sa_O2  SampleTime=t_sample  SaveFormat=Array
  wires:
  Olszowka SI units/1(P_CO2) -> To Workspace13/1
  Olszowka SI units/2(P_O2) -> To Workspace12/1
  Olszowka SI units/3(pH) -> To Workspace11/1
  C_a_gases/1 -> Demux1/1
  Demux1/2 -> Olszowka SI units/2(C_O2), To Workspace15/1
  Demux1/1 -> Olszowka SI units/1(C_CO2), To Workspace14/1
  Olszowka SI units/4(Sat) -> To Workspace16/1

== system Resp18e_updatedPulse/Patient/LV + Aorta/Cardiac mixing LV ==
  note: This block simlates mixing in the LV of the
      | heart and the ascending aorta. Time constant and
      | further detail obtained from Khoo et al (#116) and
      | Ghazanshahi & Khoo (#259)
  Cec_gases : Inport  OutDataType=sfix(16)  OutScaling=2^0
  "CO2 O2 " : Mux  Inputs=2
  CO2_LV : Integrator  InitialCondition=m_CO2_LV_b_i
  Demux : Demux  Outputs=2
  O2_LV : Integrator  InitialCondition=m_O2_LV_b_i
  P8 : Product  Inputs=**  OutDataType=sfix(16)  OutScaling=2^0  SaturateOnIntegerOverflow=on  RndMeth=Zero  InputSameDT=on  OutDataTypeStr=Inherit: Same as first input
  P9 : Product  Inputs=**  OutDataType=sfix(16)  OutScaling=2^0  SaturateOnIntegerOverflow=on  RndMeth=Zero  InputSameDT=on  OutDataTypeStr=Inherit: Same as first input
  Tidal vol4 : Sum  Inputs=-+  OutDataType=sfix(16)  OutScaling=2^0  SaturateOnIntegerOverflow=on  InputSameDT=on  OutDataTypeStr=Inherit: Same as first input
  Tidal vol5 : Sum  Inputs=+-  OutDataType=sfix(16)  OutScaling=2^0  SaturateOnIntegerOverflow=on  InputSameDT=on  OutDataTypeStr=Inherit: Same as first input
  V1_mixing : Gain  Gain=1/Vb_LV  ParameterDataType=sfix(16)  ParameterScaling=2^0  OutDataType=sfix(16)  OutScaling=2^0  SaturateOnIntegerOverflow=on  OutDataTypeStr=Inherit: Same as input  ParamDataTypeStr=Inherit: Same as input
  "V1_mixing " : Gain  Gain=1/Vb_LV  ParameterDataType=sfix(16)  ParameterScaling=2^0  OutDataType=sfix(16)  OutScaling=2^0  SaturateOnIntegerOverflow=on  OutDataTypeStr=Inherit: Same as input  ParamDataTypeStr=Inherit: Same as input
  Ca_gases : Outport  OutDataType=sfix(16)  OutScaling=2^0
  wires:
  V1_mixing/1 -> Tidal vol4/1, "CO2 O2 "/1
  Tidal vol4/1 -> P8/1
  P8/1 -> CO2_LV/1
  CO2_LV/1 -> V1_mixing/1
  P9/1 -> O2_LV/1
  Tidal vol5/1 -> P9/1
  [Qpdot] -> P8/2, P9/2
  O2_LV/1 -> "V1_mixing "/1
  "V1_mixing "/1 -> Tidal vol5/2, "CO2 O2 "/2
  Cec_gases/1 -> Demux/1
  Demux/1 -> Tidal vol4/2
  Demux/2 -> Tidal vol5/1
  "CO2 O2 "/1 -> Ca_gases/1

== system Resp18e_updatedPulse/Patient/LV + Aorta/Delay_common ==
  note: This block performs the following functions:
      | 1. Keeps a record of the quantity of CO2 in aorta
      | 2.  Keeps a record of the quantity of O2 in aorta
      | 3. Delays C_CO2 and C_O2 signals by a time
      | proportional to the aortic volume and inversely
      | proportional to Qpdot.
      | 4. Outputs are delayed C_CO2 and C_O2 signals (moles/l)
      | NB: This subsystem cannot handle varying Qpdot
  note: Constant Qpdot only
  C_gases : Inport  PortDimensions=2  OutDataType=sfix(16)  OutScaling=2^0
  CO2 O2 : Demux  Outputs=2
  CO2 xport delay : VariableTransportDelay  MaximumDelay=20  InitialOutput=C_a_CO2_i  MaximumPoints=n_delay_buffer
  CO2_d : Integrator  InitialCondition=m_CO2_common_b_i
  Fixed delay : Fcn  Expr=Vb_common/u(1)
  Mux : Mux  Inputs=2
  O2 delay : VariableTransportDelay  MaximumDelay=20  InitialOutput=C_a_O2_i  MaximumPoints=n_delay_buffer
  O2_d : Integrator  InitialCondition=m_O2_common_b_i
  Product{1..4} (4 alike) : Product  OutDataType=sfix(16)  OutScaling=2^0  SaturateOnIntegerOverflow=on  RndMeth=Zero  InputSameDT=on  OutDataTypeStr=Inherit: Same as first input
  Terminator : Terminator
  Terminator1 : Terminator
  Tidal vol2 : Sum  Inputs=+-  OutDataType=sfix(16)  OutScaling=2^0  SaturateOnIntegerOverflow=on  InputSameDT=on  OutDataTypeStr=Inherit: Same as first input
  Tidal vol3 : Sum  Inputs=+-  OutDataType=sfix(16)  OutScaling=2^0  SaturateOnIntegerOverflow=on  InputSameDT=on  OutDataTypeStr=Inherit: Same as first input
  Ca_gases_d : Outport  OutDataType=sfix(16)  OutScaling=2^0
  wires:
  Fixed delay/1 -> CO2 xport delay/2, O2 delay/2
  Tidal vol2/1 -> CO2_d/1
  Product1/1 -> Tidal vol2/1
  Tidal vol3/1 -> O2_d/1
  Product4/1 -> Tidal vol3/1
  O2_d/1 -> Terminator1/1
  CO2_d/1 -> Terminator/1
  CO2 xport delay/1 -> Product2/1, Mux/1
  O2 delay/1 -> Product3/2, Mux/2
  Product3/1 -> Tidal vol3/2
  Product2/1 -> Tidal vol2/2
  CO2 O2/1 -> Product1/1, CO2 xport delay/1
  C_gases/1 -> CO2 O2/1
  CO2 O2/2 -> O2 delay/1, Product4/2
  Mux/1 -> Ca_gases_d/1
  [Qpdot] -> Fixed delay/1, Product1/2, Product3/1, Product4/1, Product2/2

== system Resp18e_updatedPulse/Patient/Large Veins/Flow prop mix ==
  C1_gases : Inport  PortDimensions=3  OutDataType=sfix(16)  OutScaling=2^0
  C2_gases : Inport  Port=2  PortDimensions=3  OutDataType=sfix(16)  OutScaling=2^0
  Demux : Demux  Outputs=3
  Demux1 : Demux  Outputs=3
  Mux : Mux  Inputs=3
  P10 : Product  Inputs=*/  OutDataType=sfix(16)  OutScaling=2^0  SaturateOnIntegerOverflow=on  RndMeth=Zero  InputSameDT=on  OutDataTypeStr=Inherit: Same as first input
  P{4..7} (4 alike) : Product  Inputs=**  OutDataType=sfix(16)  OutScaling=2^0  SaturateOnIntegerOverflow=on  RndMeth=Zero  InputSameDT=on  OutDataTypeStr=Inherit: Same as first input
  P8 : Product  Inputs=*/  OutDataType=sfix(16)  OutScaling=2^0  SaturateOnIntegerOverflow=on  RndMeth=Zero  InputSameDT=on  OutDataTypeStr=Inherit: Same as first input
  Tidal vol4 : Sum  OutDataType=sfix(16)  OutScaling=2^0  SaturateOnIntegerOverflow=on  InputSameDT=on  OutDataTypeStr=Inherit: Same as first input
  Tidal vol5 : Sum  OutDataType=sfix(16)  OutScaling=2^0  SaturateOnIntegerOverflow=on  InputSameDT=on  OutDataTypeStr=Inherit: Same as first input
  Tidal vol6 : Sum  OutDataType=sfix(16)  OutScaling=2^0  SaturateOnIntegerOverflow=on  InputSameDT=on  OutDataTypeStr=Inherit: Same as first input
  C_gases : Outport  OutDataType=sfix(16)  OutScaling=2^0
  wires:
  Demux1/2 -> P7/1
  Demux1/1 -> P6/1
  Demux/2 -> P5/1
  Demux/1 -> P4/1
  P10/1 -> Mux/2
  Tidal vol6/1 -> P10/1
  Tidal vol5/1 -> P8/1
  Tidal vol4/1 -> P10/2, P8/2, Mux/3
  P8/1 -> Mux/1
  Demux1/3 -> P7/2, Tidal vol4/2, P6/2
  P6/1 -> Tidal vol5/2
  Demux/3 -> P5/2, P4/2, Tidal vol4/1
  P7/1 -> Tidal vol6/2
  P5/1 -> Tidal vol6/1
  P4/1 -> Tidal vol5/1
  C2_gases/1 -> Demux1/1
  C1_gases/1 -> Demux/1
  Mux/1 -> C_gases/1

== system Resp18e_updatedPulse/Patient/Large Veins/Flow prop mix1 ==
  C1_gases : Inport  PortDimensions=3  OutDataType=sfix(16)  OutScaling=2^0
  C2_gases : Inport  Port=2  PortDimensions=3  OutDataType=sfix(16)  OutScaling=2^0
  Demux : Demux  Outputs=3
  Demux1 : Demux  Outputs=3
  Mux : Mux  Inputs=3
  P10 : Product  Inputs=*/  OutDataType=sfix(16)  OutScaling=2^0  SaturateOnIntegerOverflow=on  RndMeth=Zero  InputSameDT=on  OutDataTypeStr=Inherit: Same as first input
  P{4..7} (4 alike) : Product  Inputs=**  OutDataType=sfix(16)  OutScaling=2^0  SaturateOnIntegerOverflow=on  RndMeth=Zero  InputSameDT=on  OutDataTypeStr=Inherit: Same as first input
  P8 : Product  Inputs=*/  OutDataType=sfix(16)  OutScaling=2^0  SaturateOnIntegerOverflow=on  RndMeth=Zero  InputSameDT=on  OutDataTypeStr=Inherit: Same as first input
  Tidal vol4 : Sum  OutDataType=sfix(16)  OutScaling=2^0  SaturateOnIntegerOverflow=on  InputSameDT=on  OutDataTypeStr=Inherit: Same as first input
  Tidal vol5 : Sum  OutDataType=sfix(16)  OutScaling=2^0  SaturateOnIntegerOverflow=on  InputSameDT=on  OutDataTypeStr=Inherit: Same as first input
  Tidal vol6 : Sum  OutDataType=sfix(16)  OutScaling=2^0  SaturateOnIntegerOverflow=on  InputSameDT=on  OutDataTypeStr=Inherit: Same as first input
  C_gases : Outport  OutDataType=sfix(16)  OutScaling=2^0
  wires:
  Mux/1 -> C_gases/1
  C1_gases/1 -> Demux/1
  C2_gases/1 -> Demux1/1
  P4/1 -> Tidal vol5/1
  P5/1 -> Tidal vol6/1
  P7/1 -> Tidal vol6/2
  Demux/3 -> Tidal vol4/1, P4/2, P5/2
  P6/1 -> Tidal vol5/2
  Demux1/3 -> P6/2, Tidal vol4/2, P7/2
  P8/1 -> Mux/1
  Tidal vol4/1 -> Mux/3, P8/2, P10/2
  Tidal vol5/1 -> P8/1
  Tidal vol6/1 -> P10/1
  P10/1 -> Mux/2
  Demux/1 -> P4/1
  Demux/2 -> P5/1
  Demux1/1 -> P6/1
  Demux1/2 -> P7/1
